simulink subsystem "Data_Logging"  (R2020b)
settings: Solver=VariableStepAuto  StartTime=0.0  StopTime=10.0  RelTol=1e-3
settings Model: Creator=dffleiss  LastModifiedBy=dffleiss

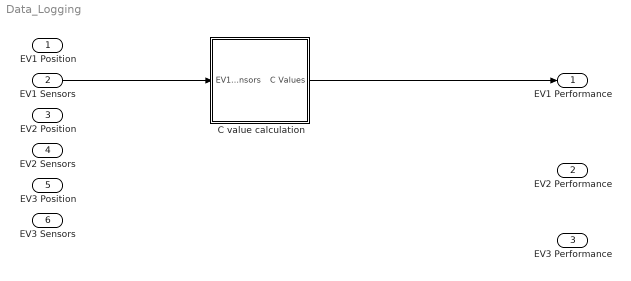
== system Data_Logging ==
  EV1 Position : Inport
  EV1 Sensors : Inport  Port=2
  EV2 Position : Inport  Port=3
  EV2 Sensors : Inport  Port=4
  EV3 Position : Inport  Port=5
  EV3 Sensors : Inport  Port=6
  C value calculation : Subsystem
  EV1 Performance : Outport
  EV2 Performance : Outport  Port=2
  EV3 Performance : Outport  Port=3
  wires:
  EV1 Sensors/1 -> C value calculation/1(EV1 Sensors)
  C value calculation/1(C Values) -> EV1 Performance/1

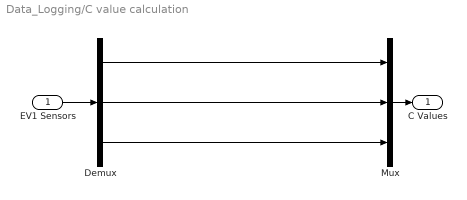
== system Data_Logging/C value calculation ==
  EV1 Sensors : Inport
  Demux : Demux  Outputs=3
  Mux : Mux  Inputs=3
  C Values : Outport
  wires:
  Mux/1 -> C Values/1
  Demux/3 -> Mux/3
  Demux/2 -> Mux/2
  Demux/1 -> Mux/1
  EV1 Sensors/1 -> Demux/1
